simulink model "Model1angular"  (R2014b)
settings: Solver=ode45  StartTime=0.0  StopTime=100.0  RelTol=1e-4
values from neighbouring files (symbols this model uses):
  A = [-1 Sr1 1 0 0 0; 0 -1 0 1 0 0; -1 Sr2 0 0 1 0; 0 -1 0 0 0 1]    [Internalforce_symbolic.m]    (also in Model1Init.m = [-eye(3),eye(3),zeros(3);-eye(3),zeros(3),eye(3)])
  d1 = 5    [Model1Init.m]
  d2 = 5    [Model1Init.m]
  g = [0;0;-9.81]    [Model1Init.m]
  G_Mplus = [m1/m0 *eye(3);m2/m0 *eye(3)]    [Model1Init.m]
  k1 = 1    [Model1Init.m]
  k2 = 1    [Model1Init.m]
  m0 = 20    [Model1Init.m]
  m1 = 10    [Model1Init.m]
  m2 = 10    [Model1Init.m]
  r = [1 0 0;-1 0 0]    [Model1Init.m]
undefined symbols (not defined in the file or in its folder): delta1, delta2, j0, j1, j2, kappa1, kappa2
libraries: aerolibtransform2 x4, aerolibutil x2, dspinverses x2
settings Model: Creator=Martin  LastModifiedBy=Martin

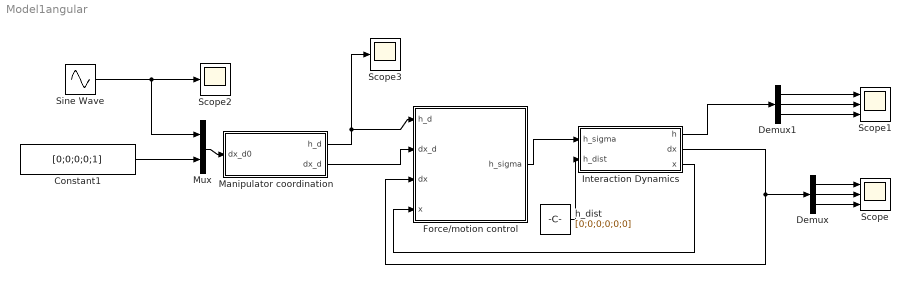
== system Model1angular ==
  Constant1 : Constant  Value=[0;0;0;0;1]
  Demux : Demux  Outputs=3
  Demux1 : Demux  Outputs=3
  Force/motion control : Subsystem
  Interaction Dynamics : Subsystem
  Manipulator coordination : Subsystem
  Mux : Mux  Inputs=2
  Scope : Scope  NumInputPorts=3
      settings: ShowLegends=on  YMin=-5~-5~-5  YMax=5~5~5
  Scope1 : Scope  NumInputPorts=3
      settings: ShowLegends=on  YMin=-50~-100~-100  YMax=200~20~20
  Scope2 : Scope
      settings: SaveName=ScopeData2
  Scope3 : Scope
      settings: SaveName=ScopeData5
  Sine Wave : Sin  SampleTime=0
  h_dist : Constant  Value=[0;0;0;0;0;0]
  wires:
  Interaction Dynamics/2(dx) -> Force/motion control/3(dx), Demux/1
  Demux/1 -> Scope/1
  Demux/2 -> Scope/2
  Demux/3 -> Scope/3
  Force/motion control/1(h_sigma) -> Interaction Dynamics/1(h_sigma)
  Manipulator coordination/2(dx_d) -> Force/motion control/2(dx_d)
  Interaction Dynamics/1(h) -> Demux1/1
  Demux1/1 -> Scope1/1
  Demux1/2 -> Scope1/2
  Demux1/3 -> Scope1/3
  h_dist/1 -> Interaction Dynamics/2(h_dist)
  Manipulator coordination/1(h_d) -> Force/motion control/1(h_d), Scope3/1
  Mux/1 -> Manipulator coordination/1(dx_d0)
  Constant1/1 -> Mux/2
  Sine Wave/1 -> Scope2/1, Mux/1
  Interaction Dynamics/3(x) -> Force/motion control/4(x)

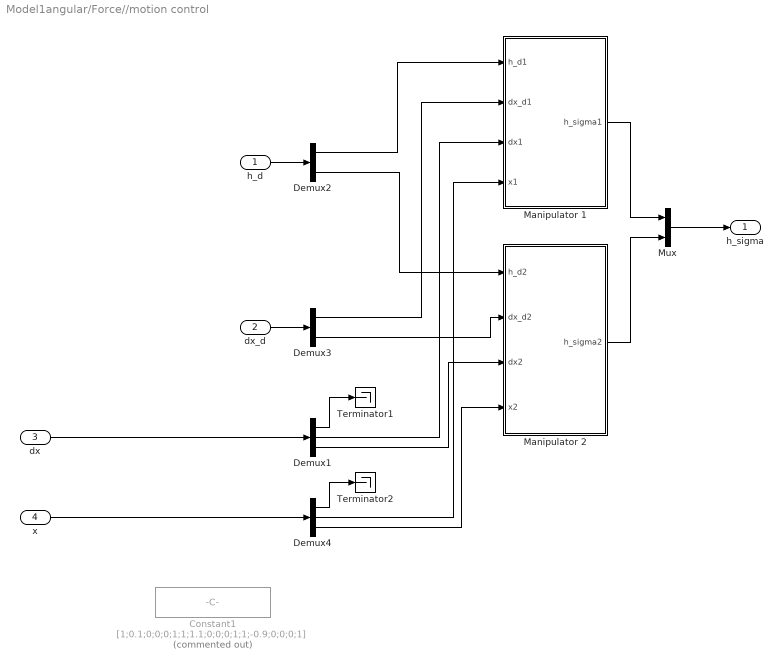
== system Model1angular/Force//motion control ==
  h_d : Inport
  dx_d : Inport  Port=2
  dx : Inport  Port=3
  x : Inport  Port=4
  Constant1 : Constant  Commented=on  Value=[1;0.1;0;0;0;1;1;1.1;0;0;0;1;1;-0.9;0;0;0;1]
  Demux1 : Demux  Outputs=3
  Demux2 : Demux  Outputs=2
  Demux3 : Demux  Outputs=2
  Demux4 : Demux  Outputs=3
  Manipulator 1 : Subsystem
  Manipulator 2 : Subsystem
  Mux : Mux  Inputs=2
  Terminator1 : Terminator
  Terminator2 : Terminator
  h_sigma : Outport
  wires:
  Manipulator 1/1(h_sigma1) -> Mux/1
  Manipulator 2/1(h_sigma2) -> Mux/2
  Mux/1 -> h_sigma/1
  Demux1/3 -> Manipulator 2/3(dx2)
  Demux1/2 -> Manipulator 1/3(dx1)
  Demux1/1 -> Terminator1/1
  dx_d/1 -> Demux3/1
  h_d/1 -> Demux2/1
  Demux2/1 -> Manipulator 1/1(h_d1)
  Demux2/2 -> Manipulator 2/1(h_d2)
  Demux3/1 -> Manipulator 1/2(dx_d1)
  Demux3/2 -> Manipulator 2/2(dx_d2)
  dx/1 -> Demux1/1
  x/1 -> Demux4/1
  Demux4/1 -> Terminator2/1
  Demux4/2 -> Manipulator 1/4(x1)
  Demux4/3 -> Manipulator 2/4(x2)

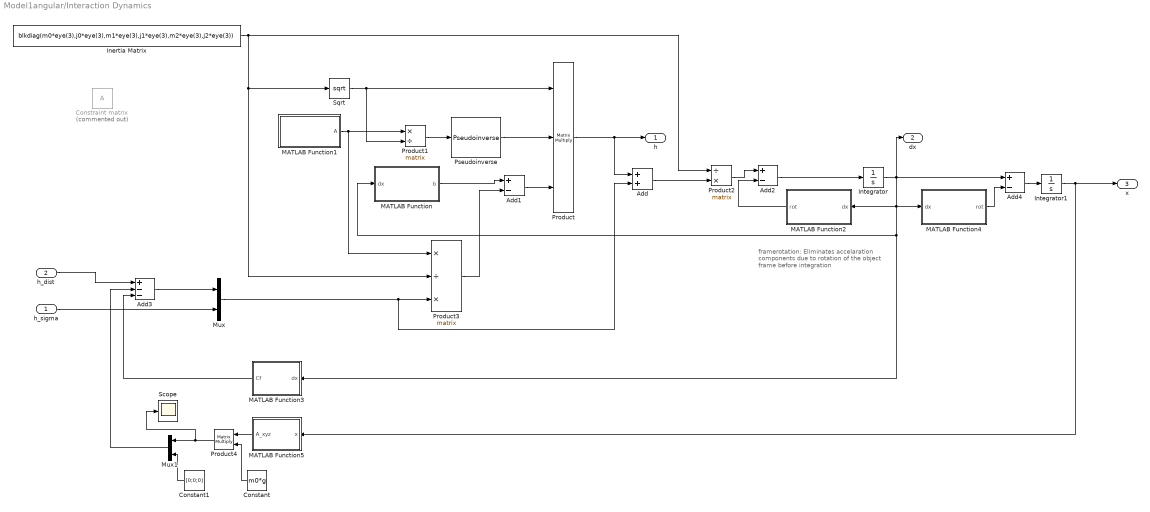
== system Model1angular/Interaction Dynamics ==
  note: framerotation: Eliminates accelaration
      |  components  due to rotation of the
      |  object frame before integration
  h_sigma : Inport
  h_dist : Inport  Port=2
  Add : Sum
  Add1 : Sum  Inputs=+-
  Add2 : Sum  Inputs=+-
  Add3 : Sum  Inputs=+--
  Add4 : Sum  Inputs=+-
  Constant : Constant  Value=m0*g
  Constant1 : Constant  Value=[0;0;0]
  Constraint matrix : Constant  Commented=on  Value=A
  Inertia Matrix : Constant  Value=blkdiag(m0*eye(3),j0*eye(3),m1*eye(3),j1*eye(3),m2*eye(3),j2*eye(3))
  Integrator : Integrator
  Integrator1 : Integrator
  MATLAB Function : MATLAB Function  TreatAsAtomicUnit=on
  MATLAB Function1 : MATLAB Function  TreatAsAtomicUnit=on
  MATLAB Function2 : MATLAB Function  TreatAsAtomicUnit=on
  MATLAB Function3 : MATLAB Function  TreatAsAtomicUnit=on
  MATLAB Function4 : MATLAB Function  TreatAsAtomicUnit=on
  MATLAB Function5 : MATLAB Function  TreatAsAtomicUnit=on
  Mux : Mux  Inputs=2
  Mux1 : Mux  Inputs=2
  Product : Product  Inputs=***  Multiplication=Matrix(*)
  Product1 : Product  Inputs=*/  Multiplication=Matrix(*)
  Product2 : Product  Inputs=/*  Multiplication=Matrix(*)
  Product3 : Product  Inputs=*/*  Multiplication=Matrix(*)
  Product4 : Product  Multiplication=Matrix(*)
  Pseudoinverse : dspinverses/Pseudoinverse  wanterr=off
  Scope : Scope
      settings: ShowLegends=on  SaveName=ScopeData6
  Sqrt : Sqrt  SaturateOnIntegerOverflow=on
  h : Outport
  dx : Outport  Port=2
  x : Outport  Port=3
  wires:
  Sqrt/1 -> Product/1, Product1/2
  Pseudoinverse/1 -> Product/2
  Product1/1 -> Pseudoinverse/1
  Integrator/1 -> dx/1, Add4/1, MATLAB Function4/1(dx), MATLAB Function2/1(dx), MATLAB Function3/1(dx), MATLAB Function/1(dx)
  Product/1 -> h/1, Add/1
  Add/1 -> Product2/2
  Inertia Matrix/1 -> Product2/1, Sqrt/1, Product3/2
  h_sigma/1 -> Mux/2
  Add1/1 -> Product/3
  MATLAB Function/1(b) -> Add1/1
  Product3/1 -> Add1/2
  Mux/1 -> Add/2, Product3/3
  MATLAB Function1/1(A) -> Product1/1, Product3/1
  Product2/1 -> Add2/1
  Add2/1 -> Integrator/1
  MATLAB Function2/1(rot) -> Add2/2
  Add3/1 -> Mux/1
  h_dist/1 -> Add3/1
  Integrator1/1 -> MATLAB Function5/1(x), x/1
  Add4/1 -> Integrator1/1
  MATLAB Function4/1(rot) -> Add4/2
  MATLAB Function5/1(A_xyz) -> Product4/1
  MATLAB Function3/1(Cf) -> Add3/3
  Constant/1 -> Product4/2
  Product4/1 -> Scope/1, Mux1/1
  Constant1/1 -> Mux1/2
  Mux1/1 -> Add3/2

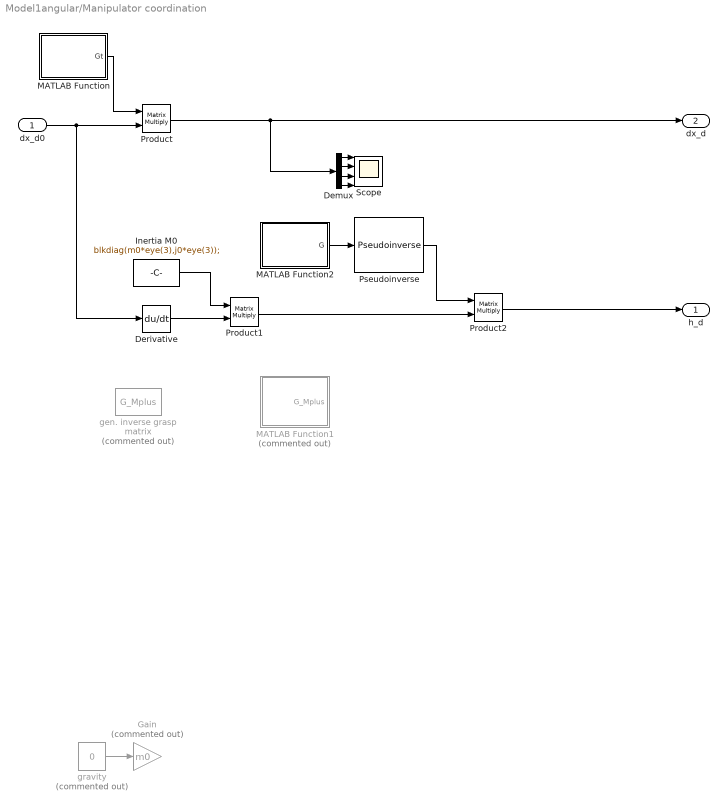
== system Model1angular/Manipulator coordination ==
  dx_d0 : Inport
  Demux : Demux
  Derivative : Derivative
  Gain : Gain  Commented=on  Gain=m0
  Inertia M0 : Constant  Value=blkdiag(m0*eye(3),j0*eye(3));
  MATLAB Function : MATLAB Function  TreatAsAtomicUnit=on
  MATLAB Function1 : MATLAB Function  Commented=on  TreatAsAtomicUnit=on
  MATLAB Function2 : MATLAB Function  TreatAsAtomicUnit=on
  Product : Product  Multiplication=Matrix(*)
  Product1 : Product  Multiplication=Matrix(*)
  Product2 : Product  Multiplication=Matrix(*)
  Pseudoinverse : dspinverses/Pseudoinverse  wanterr=off
  Scope : Scope  NumInputPorts=4
      settings: ShowLegends=on  YMin=-5~-5~-5~-5  YMax=5~5~5~5  SaveName=ScopeData3
  gen. inverse grasp matrix : Constant  Commented=on  Value=G_Mplus
  gravity : Constant  Commented=on  Value=0
  h_d : Outport
  dx_d : Outport  Port=2
  wires:
  dx_d0/1 -> Derivative/1, Product/2
  MATLAB Function/1(Gt) -> Product/1
  Product/1 -> Demux/1, dx_d/1
  Derivative/1 -> Product1/2
  gravity/1 -> Gain/1
  Product1/1 -> Product2/2
  Product2/1 -> h_d/1
  Demux/1 -> Scope/1
  Demux/2 -> Scope/2
  Demux/3 -> Scope/3
  Demux/4 -> Scope/4
  Inertia M0/1 -> Product1/1
  MATLAB Function2/1(G) -> Pseudoinverse/1
  Pseudoinverse/1 -> Product2/1

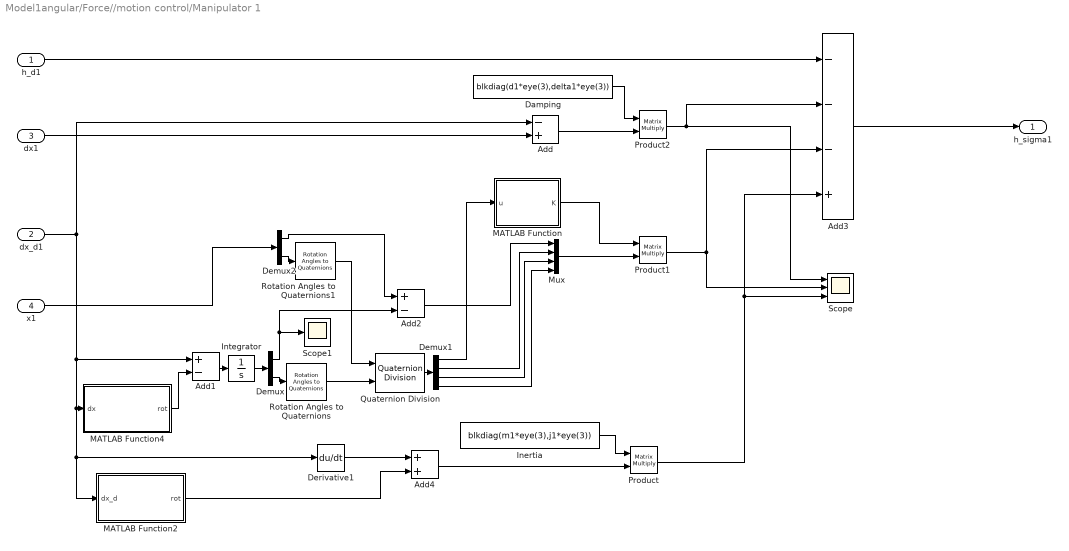
== system Model1angular/Force//motion control/Manipulator 1 ==
  h_d1 : Inport
  dx_d1 : Inport  Port=2
  dx1 : Inport  Port=3
  x1 : Inport  Port=4
  Add : Sum  Inputs=-+
  Add1 : Sum  Inputs=+-
  Add2 : Sum  Inputs=+-
  Add3 : Sum  Inputs=---+
  Add4 : Sum
  Damping : Constant  Value=blkdiag(d1*eye(3),delta1*eye(3))
  Demux : Demux  Outputs=2
  Demux1 : Demux
  Demux2 : Demux  Outputs=2
  Derivative1 : Derivative
  Inertia : Constant  Value=blkdiag(m1*eye(3),j1*eye(3))
  Integrator : Integrator
  MATLAB Function : MATLAB Function  TreatAsAtomicUnit=on
  MATLAB Function2 : MATLAB Function  TreatAsAtomicUnit=on
  MATLAB Function4 : MATLAB Function  TreatAsAtomicUnit=on
  Mux : Mux
  Product : Product  Multiplication=Matrix(*)
  Product1 : Product  Multiplication=Matrix(*)
  Product2 : Product  Multiplication=Matrix(*)
  Quaternion Division : aerolibutil/Quaternion Division
  Rotation Angles to Quaternions : aerolibtransform2/Rotation Angles to Quaternions  rotationOrder=XYZ
  Rotation Angles to Quaternions1 : aerolibtransform2/Rotation Angles to Quaternions  rotationOrder=XYZ
  Scope : Scope  NumInputPorts=3
      settings: ShowLegends=on  YMin=-5~-5~-5  YMax=5~5~5  SaveName=ScopeData4
  Scope1 : Scope
      settings: ShowLegends=on  SaveName=ScopeData7
  h_sigma1 : Outport
  wires:
  dx_d1/1 -> Add1/1, Derivative1/1, MATLAB Function2/1(dx_d), MATLAB Function4/1(dx), Add/1
  Mux/1 -> Product1/2
  Add/1 -> Product2/2
  Damping/1 -> Product2/1
  Inertia/1 -> Product/1
  Product/1 -> Scope/3, Add3/4
  h_d1/1 -> Add3/1
  Add3/1 -> h_sigma1/1
  Integrator/1 -> Demux/1
  Demux/2 -> Rotation Angles to Quaternions/1
  dx1/1 -> Add/2
  x1/1 -> Demux2/1
  Demux2/2 -> Rotation Angles to Quaternions1/1
  MATLAB Function/1(K) -> Product1/1
  Rotation Angles to Quaternions1/1 -> Quaternion Division/1
  Rotation Angles to Quaternions/1 -> Quaternion Division/2
  Quaternion Division/1 -> Demux1/1
  Demux1/1 -> MATLAB Function/1(u)
  Demux2/1 -> Add2/1
  Demux/1 -> Scope1/1, Add2/2
  Add2/1 -> Mux/1
  Demux1/2 -> Mux/2
  Demux1/3 -> Mux/3
  Demux1/4 -> Mux/4
  Product2/1 -> Scope/1, Add3/2
  Product1/1 -> Add3/3, Scope/2
  MATLAB Function4/1(rot) -> Add1/2
  Add1/1 -> Integrator/1
  Add4/1 -> Product/2
  Derivative1/1 -> Add4/1
  MATLAB Function2/1(rot) -> Add4/2

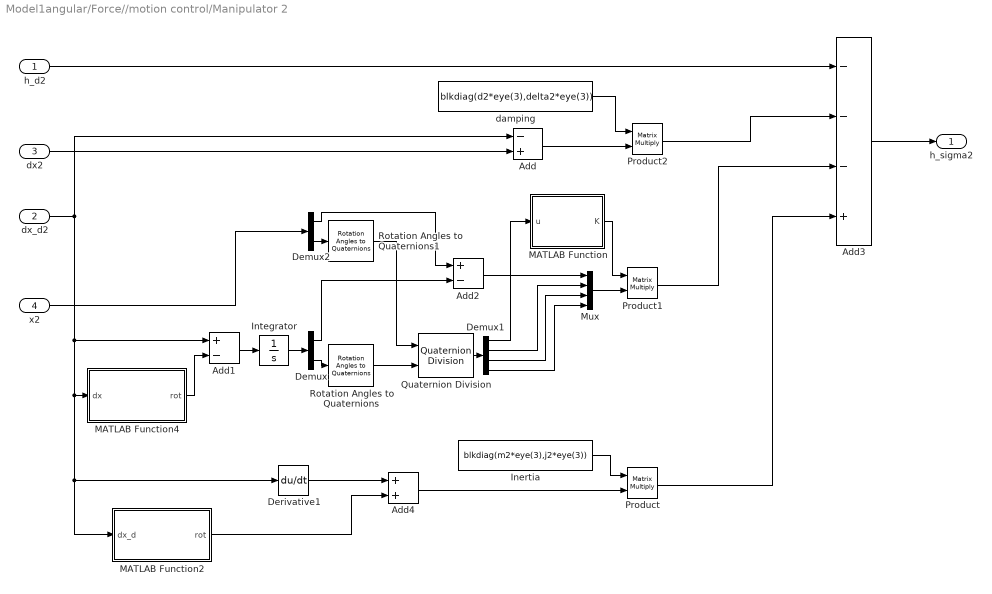
== system Model1angular/Force//motion control/Manipulator 2 ==
  h_d2 : Inport
  dx_d2 : Inport  Port=2
  dx2 : Inport  Port=3
  x2 : Inport  Port=4
  Add : Sum  Inputs=-+
  Add1 : Sum  Inputs=+-
  Add2 : Sum  Inputs=+-
  Add3 : Sum  Inputs=---+
  Add4 : Sum
  Demux : Demux  Outputs=2
  Demux1 : Demux
  Demux2 : Demux  Outputs=2
  Derivative1 : Derivative
  Inertia : Constant  Value=blkdiag(m2*eye(3),j2*eye(3))
  Integrator : Integrator
  MATLAB Function : MATLAB Function  TreatAsAtomicUnit=on
  MATLAB Function2 : MATLAB Function  TreatAsAtomicUnit=on
  MATLAB Function4 : MATLAB Function  TreatAsAtomicUnit=on
  Mux : Mux
  Product : Product  Multiplication=Matrix(*)
  Product1 : Product  Multiplication=Matrix(*)
  Product2 : Product  Multiplication=Matrix(*)
  Quaternion Division : aerolibutil/Quaternion Division
  Rotation Angles to Quaternions : aerolibtransform2/Rotation Angles to Quaternions  rotationOrder=XYZ
  Rotation Angles to Quaternions1 : aerolibtransform2/Rotation Angles to Quaternions  rotationOrder=XYZ
  damping : Constant  Value=blkdiag(d2*eye(3),delta2*eye(3))
  h_sigma2 : Outport
  wires:
  dx_d2/1 -> Add/1, Add1/1, Derivative1/1, MATLAB Function2/1(dx_d), MATLAB Function4/1(dx)
  dx2/1 -> Add/2
  Add/1 -> Product2/2
  damping/1 -> Product2/1
  Inertia/1 -> Product/1
  Product/1 -> Add3/4
  h_d2/1 -> Add3/1
  Add3/1 -> h_sigma2/1
  Integrator/1 -> Demux/1
  Demux/2 -> Rotation Angles to Quaternions/1
  x2/1 -> Demux2/1
  Demux2/2 -> Rotation Angles to Quaternions1/1
  MATLAB Function/1(K) -> Product1/1
  Mux/1 -> Product1/2
  Rotation Angles to Quaternions/1 -> Quaternion Division/2
  Rotation Angles to Quaternions1/1 -> Quaternion Division/1
  Quaternion Division/1 -> Demux1/1
  Demux1/1 -> MATLAB Function/1(u)
  Add2/1 -> Mux/1
  Demux2/1 -> Add2/1
  Demux/1 -> Add2/2
  Demux1/2 -> Mux/2
  Demux1/3 -> Mux/3
  Demux1/4 -> Mux/4
  Product2/1 -> Add3/2
  Product1/1 -> Add3/3
  Add1/1 -> Integrator/1
  MATLAB Function4/1(rot) -> Add1/2
  MATLAB Function2/1(rot) -> Add4/2
  Add4/1 -> Product/2
  Derivative1/1 -> Add4/1

== matlab function Model1angular/Force//motion control/Manipulator 2/MATLAB Function ==
  data: u input; K output; k2 parameter; kappa2 parameter
function K = stiffness(u,k2,kappa2)
K = blkdiag(k2*eye(3),2*u*kappa2*eye(3));

== matlab function Model1angular/Force//motion control/Manipulator 1/MATLAB Function ==
  data: u input; K output; k1 parameter; kappa1 parameter
function K = stiffness(u,k1,kappa1)
K = blkdiag(k1*eye(3),2*u*kappa1*eye(3));

== matlab function Model1angular/Interaction Dynamics/MATLAB Function ==
  data: dx input; b output; r parameter
function b = constraintvector(dx,r)
b = [(dx(4:6)'*r(1:3))*dx(4:6)-(dx(4:6)'*dx(4:6))*r(1:3);
    zeros(3,1);
    (dx(4:6)'*r(4:6))*dx(4:6)-(dx(4:6)'*dx(4:6))*r(4:6);
    zeros(3,1)];

== matlab function Model1angular/Manipulator coordination/MATLAB Function ==
  data: r parameter; Gt output
function Gt = GraspMatrix(r)
Gt = [eye(3) zeros(3) eye(3) zeros(3); skew_sm(r(1:3)) eye(3) skew_sm(r(4:6)) eye(3)]';

== matlab function Model1angular/Interaction Dynamics/MATLAB Function1 ==
  data: r parameter; A output
function A = constraintMatrix(r)
A = [-eye(3),skew_sm(r(1:3)),eye(3),zeros(3,9);
    zeros(3),-eye(3),zeros(3),eye(3),zeros(3,6);
    -eye(3),skew_sm(r(4:6)),zeros(3,6),eye(3),zeros(3);
    zeros(3),-eye(3),zeros(3,9),eye(3)];

== matlab function Model1angular/Manipulator coordination/MATLAB Function1 ==
  data: r parameter; G_Mplus output; m0 parameter; m1 parameter; m2 parameter; j0 parameter; j1 parameter; j2 parameter
function G_Mplus = geninvGraspM(r,m0,m1,m2,j0,j1,j2)
G_Mplus = [m1/m0*eye(3) (m1/j0*skew_sm(r(1:3)))';
    zeros(3) j1/j0*eye(3);
    m2/m0*eye(3) (m2/j0*skew_sm(r(4:6)))';
    zeros(3) j2/j0*eye(3)];

== matlab function Model1angular/Interaction Dynamics/MATLAB Function2 ==
  data: dx input; rot output; r parameter
function rot = framerotation(dx,r)
rot = [zeros(6,1);
    (dx(4:6)'*r(1:3))*dx(4:6)-(dx(4:6)'*dx(4:6))*r(1:3);
    zeros(3,1);
    (dx(4:6)'*r(4:6))*dx(4:6)-(dx(4:6)'*dx(4:6))*r(4:6);
    zeros(3,1)];

== matlab function Model1angular/Interaction Dynamics/MATLAB Function3 ==
  data: dx input; Cf output; j0 parameter
function Cf = CoriolisF(dx,j0)
Cf = [zeros(3,1);
      j0*skew_sm(dx(4:6))*dx(4:6)];

== matlab function Model1angular/Manipulator coordination/MATLAB Function2 ==
  data: r parameter; G output
function G = GraspMatrix(r)
G = [eye(3) zeros(3) eye(3) zeros(3); skew_sm(r(1:3)) eye(3) skew_sm(r(4:6)) eye(3)];

== matlab function Model1angular/Interaction Dynamics/MATLAB Function4 ==
  data: dx input; rot output; r parameter
function rot = framerotation(dx,r)
rot = [zeros(6,1);
    skew_sm(dx(4:6))*r(1:3);
    zeros(3,1);
    skew_sm(dx(4:6))*r(4:6);
    zeros(3,1)];

== matlab function Model1angular/Force//motion control/Manipulator 2/MATLAB Function4 ==
  data: dx input; rot output; r parameter
function rot = framerotation(dx,r)
rot = [skew_sm(dx(4:6))*r(4:6);
    zeros(3,1)];

== matlab function Model1angular/Force//motion control/Manipulator 1/MATLAB Function4 ==
  data: dx input; rot output; r parameter
function rot = framerotation(dx,r)
rot = [skew_sm(dx(4:6))*r(1:3);
    zeros(3,1)];

== matlab function Model1angular/Force//motion control/Manipulator 1/MATLAB Function2 ==
  data: dx_d input; rot output; r parameter
function rot = framerotation(dx_d,r)
rot = [(dx_d(4:6)'*r(1:3))*dx_d(4:6)-(dx_d(4:6)'*dx_d(4:6))*r(1:3);
    zeros(3,1)];

== matlab function Model1angular/Force//motion control/Manipulator 2/MATLAB Function2 ==
  data: dx_d input; rot output; r parameter
function rot = framerotation(dx_d,r)
rot = [(dx_d(4:6)'*r(4:6))*dx_d(4:6)-(dx_d(4:6)'*dx_d(4:6))*r(4:6);
    zeros(3,1)];

== matlab function Model1angular/Interaction Dynamics/MATLAB Function5 ==
  data: x input; A_xyz output
function A_xyz = rotationMatrix(x)
A_xyz = [cos(x(5))*cos(x(6)) cos(x(4))*sin(x(6))+sin(x(4))*sin(x(5))*cos(x(6)) sin(x(4))*sin(x(6))-cos(x(4))*sin(x(5))*cos(x(6));
         -cos(x(5))*sin(x(6)) cos(x(4))*cos(x(6))-sin(x(4))*sin(x(5))*sin(x(6)) sin(x(4))*cos(x(6))+cos(x(4))*sin(x(5))*sin(x(6));
         -sin(x(4)) -sin(x(4))*cos(x(5)) cos(x(4))*cos(x(5))];
